simulink model "dfig"  (R2016a)
settings: Solver=VariableStepAuto  StartTime=0.0  StopTime=2  RelTol=1e-3
model workspace (MATLAB code in the model file):
  | Rs=1;
  | Vs=220;
  | fs=60;
  | p=2;
  | T=1e-4;
  | Ts=1e-5;
  | 
  | Ls=0.2010;
  | Rr=3.122;
  | Lr=0.2010;
  | Lm=0.1917;
  | 
  | Ps=3e3;
values from neighbouring files (symbols this model uses):
  dLm = delta(1)    [fitness.m]
  dRr = delta(2)    [fitness.m]
  Nu = 10    [fitness.m]
  Ny = 20    [fitness.m]
  StepFinal = [3,3]    [fitness.m]
  StepInit = [1,1]    [fitness.m]
  StepTime = [1,1.5]    [fitness.m]
  Variac = 120    [fitness.m]
  Wup = zeros(2*Nu,2*Nu)    [fitness.m]
  Wyp = zeros(2*Ny,2*Ny)    [fitness.m]
undefined symbols (not defined in the file or in its folder): DiscIntNeverNeededParam
libraries: powerlib x9, simulink x4, simulink_extras x3, dspfdesign x1
settings Model: Creator=Lucas  LastModifiedBy=lucas
settings SolverCC: ShapePreserveControl=EnableAll  ZeroCrossControl=DisableAll
settings DataIOCC: SignalLogging=off  DSMLogging=off

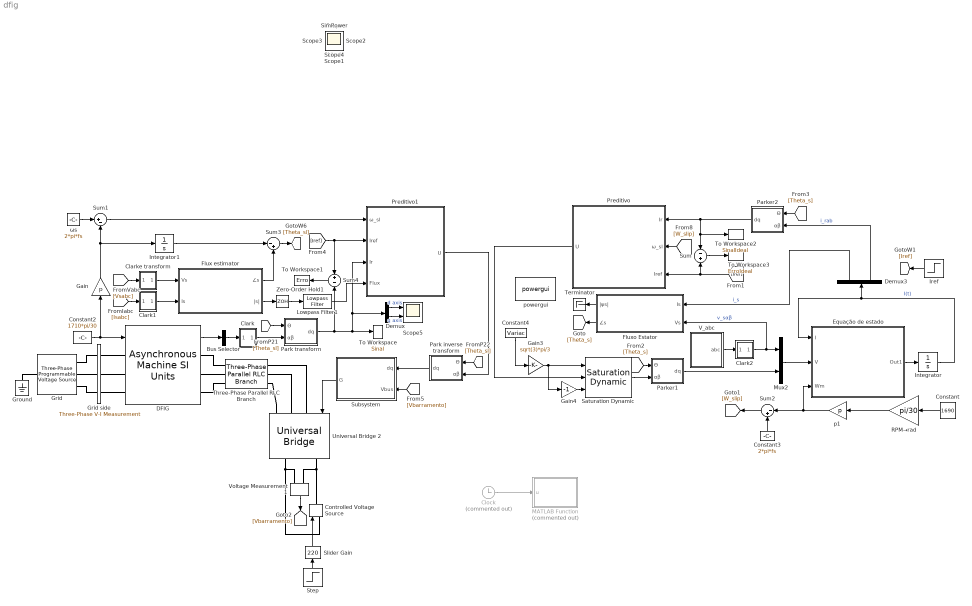
== system dfig ==
  Bus Selector : BusSelector  OutputSignals=Rotor measurements.Rotor current ir_a (A),Rotor measurements.Rotor current ir_b (A),Rotor measurements.Rotor current ir_c (A)  OutputAsBus=on
  Clark : Subsystem
      mask Display:
      | plot([0 1],[-1 0])
      | port_label('input',1,'3');
      | port_label('output', 1, '2', 'texmode', 'on')
  Clark1 : Subsystem
      mask Display:
      | plot([0 1],[-1 0])
      | port_label('input',1,'3');
      | port_label('output', 1, '2', 'texmode', 'on')
  Clark2 : Subsystem
      mask Display:
      | plot([0 1],[-1 0])
      | port_label('input',1,'3');
      | port_label('output', 1, '2', 'texmode', 'on')
  Clarke transform : Subsystem
      mask Display:
      | plot([0 1],[-1 0])
      | port_label('input',1,'3');
      | port_label('output', 1, '2', 'texmode', 'on')
  Clock : Clock  Commented=on
  Constant : Constant  Value=1690
  Constant2 : Constant  Value=1710*pi/30
      mask Display: disp('\fontsize{12}\omega_m','texmode','on')
  Constant3 : Constant  Value=2*pi*fs
      mask Display: disp('\omega_s','texmode','on')
  Constant4 : Constant  Value=Variac
  Controlled Voltage Source : powerlib/Electrical Sources/Controlled Voltage Source  Initialize=on  Source_Type=AC  Amplitude=0  Phase=0  Frequency=0  Measurements=None
  DFIG : powerlib/Machines/Asynchronous Machine SI Units  RotorType=Wound  PresetModel=No  MechanicalLoad=Speed w  ShowDetailedParameters=on  ReferenceFrame=Stationary  Units=SI  MeasurementBus=off  NominalParameters=[Ps Vs fs]  Stator=[Rs (Ls-Lm)]  Rotor=[Rr*(1+dRr/100) (Lr-Lm)]  Cage1=[0.4155 0.002066]  Cage2=[0.4168 0.0003495]  Lm=Lm*(1+dLm/100)  Mechanical=[0.05 0.005879 2]  PolePairs=p  InitialConditions=[0 0 0 0 0 0 0 0]  SimulateSaturation=off  Saturation=[14.03593122, 27.81365428, 53.79336849, 72.68890987, 97.98006896, 148.6815601, 215.7428561, 302.9841135, 428.7778367 ; 230, 322, 414, 460, 506, 552, 598, 644, 690]  LoadFlowParameters=1492000  TsPowergui=0  TsBlock=-1  IterativeModel=Trapezoidal non iterative  IterativeDiscreteModel=Trapezoidal non iterative  Pmec=0
  Demux : Demux  Outputs=2
  Demux3 : Demux  Outputs=2
  Equação de estado : Subsystem
      mask Display:
      | disp('\fontsize{16}A\cdotI(t)+B\cdotV(t)', 'texmode', 'on')
      | port_label('input', 1, 'I', 'texmode', 'on')
      | port_label('input', 2, 'V', 'texmode', 'on')
      | port_label('input', 3, '\omega_{m}', 'texmode', 'on')
      | port_label('output', 1, '\deltai(t)', 'texmode', 'on')
  Flux estimator : Subsystem
      mask Display:
      | disp('\fontsize{14}Flux Estimator', 'texmode', 'on')
      | port_label('output', 1, '\theta_s', 'texmode', 'on')
      | port_label('output', 2, '|\lambda_s|', 'texmode', 'on')
      | port_label('input', 1, 'v_s', 'texmode', 'on')
      | port_label('input', 2, 'i_s', 'texmode', 'on')
  Fluxo Estator : Subsystem
      mask Display:
      | disp('\fontsize{14}\lambda_s=\int(v_s-R_s\cdot i_s)dt', 'texmode', 'on')
      | port_label('output', 1, '|\lambda_s|', 'texmode', 'on')
      | port_label('output', 2, '\theta_s', 'texmode', 'on')
      | port_label('input', 2, 'v_s', 'texmode', 'on')
      | port_label('input', 1, 'i_s', 'texmode', 'on')
  Gain : Gain  Gain=p
  Gain3 : Gain  Gain=sqrt(3)*pi/3
  Gain4 : Gain  Gain=-1
  Grid : powerlib/Electrical Sources/Three-Phase Programmable Voltage Source  PositiveSequence="[220*sqrt(3)  0 60]"  VariationEntity=None  VariationType=Table of time-amplitude pairs  VariationTypeAlt=Step  VariationStep=0.5  VariationRate=[10]  VariationMagnitude=0.3  VariationFrequency=2  VariationTiming=[1 2]  VariationPhaseA=off  Amplitudes=[1 0.8 1.2 1.0]  TimeValues=[0 0.1 0.15 0.2]  HarmonicGeneration=off  HarmonicA=[3 0.2 -25 0]  HarmonicB=[2 0.15 35 2]  Timing="[0.05  3]"  BusType=swing  Pref=0  Qref=0  Qmin=-inf  Qmax=inf
  Grid side : powerlib/Measurements/Three-Phase V-I Measurement  VoltageMeasurement=phase-to-ground  SetLabelV=on  LabelV=Vsabc  Vpu=off  VpuLL=off  CurrentMeasurement=yes  SetLabelI=on  LabelI=Isabc  Ipu=off  Pbase=100e6  Vbase=500e3  OutputType=Complex  PhasorSimulation=off  PSBequivalent=0
  Ground : powerlib/Elements/Ground  LConnTagsString=a
  Integrator : Integrator  LimitOutput=on  UpperSaturationLimit=1e5  LowerSaturationLimit=-1e5
  Integrator1 : Integrator
  Iref : Step  Time=StepTime  Before=StepInit  After=StepFinal  SampleTime=0
  Lowpass Filter1 : dspfdesign/Lowpass Filter  FilterType=IIR  DesignForMinimumOrder=on  FilterOrder=50  PassbandFrequency=1e1  StopbandFrequency=1e2  PassbandRipple=0.1  StopbandAttenuation=80  InheritSampleRate=on  SampleRate=1e3  roundingMode=Floor  coeffsDataTypeStr=fixdt(1,16)  SimulateUsing=Interpreted execution
  MATLAB Function : MATLAB Function  Commented=on  TreatAsAtomicUnit=on
  Mux2 : Mux  Inputs=2
  Park inverse transform : Subsystem
      mask Display:
      | port_label('input', 2, 'x', 'texmode', 'on')
      | port_label('input', 1, '\theta', 'texmode', 'on')
      | port_label('output', 1, '\fontsize{14}xe^{ j\theta }', 'texmode', 'on')
  Park transform : Subsystem
      mask Display:
      | port_label('input', 2, 'x', 'texmode', 'on')
      | port_label('input', 1, '\theta', 'texmode', 'on')
      | port_label('output', 1, '\fontsize{14}xe^{ -j\theta} ', 'texmode', 'on')
  Parker1 : Subsystem
      mask Display:
      | port_label('input', 2, 'x', 'texmode', 'on')
      | port_label('input', 1, '\theta', 'texmode', 'on')
      | port_label('output', 1, '\fontsize{14}xe^{ j\theta }', 'texmode', 'on')
  Parker2 : Subsystem
      mask Display:
      | port_label('input', 2, 'x', 'texmode', 'on')
      | port_label('input', 1, '\theta', 'texmode', 'on')
      | port_label('output', 1, '\fontsize{14}xe^{ -j\theta }', 'texmode', 'on')
  Preditivo : Subsystem
      mask Display:
      | disp('\fontsize{14}Preditivo','texmode','on')
      | port_label('input', 1, 'i_{r dq} ', 'texmode', 'on')
      | port_label('input', 2, '\omega_{slip} ', 'texmode', 'on')
      | port_label('input', 3, 'i_{r ref}', 'texmode', 'on')
      | %port_label('input', 5, 'v_{r dq}', 'texmode', 'on')
      | port_label('output', 1, 'v_{r dq}', 'texmode', 'on')
  Preditivo1 : Subsystem
      mask Display:
      | disp('\fontsize{14}Predictive\newlineController','texmode','on')
      | port_label('input', 3, 'y(k)', 'texmode', 'on')
      | port_label('input', 4, '\lambda(k)', 'texmode', 'on')
      | port_label('input', 1, '\omega_{sl} ', 'texmode', 'on')
      | port_label('input', 2, 'y_{ref} (k)', 'texmode', 'on')
      | port_label('output', 1, 'u(k)', 'texmode', 'on')
  RPM→rad : Gain  Gain=pi/30
  Saturation Dynamic : simulink/Discontinuities/Saturation Dynamic  OutMin=[]  OutMax=[]  OutDataTypeStr=Inherit: Same as second input  OutDataType=fixdt(1, 16)  OutScaling=2^-10  DoSatur=off
  Scope5 : Scope  NumInputPorts=2
  Slider Gain : simulink/Math Operations/Slider Gain  low=1  gain=220  high=440
  Step : Step  Time=0  Before=1e-4  SampleTime=0
  Subsystem : Subsystem
      mask Display:
      | disp('\fontsize{14}SVPWM','texmode','on')
      | 
      | port_label('input', 1, 'dq', 'texmode', 'on')
      | port_label('input', 2, 'V_{bus}', 'texmode', 'on')
      | 
      | port_label('output', 1, 'G', 'texmode', 'on')
  Sum : Sum  Inputs=-|+
  Sum1 : Sum  Inputs=|+-
  Sum2 : Sum  Inputs=|-+
  Sum3 : Sum  Inputs=|-+
  Sum4 : Sum  Inputs=+|-
  Terminator : Terminator
  Three-Phase Parallel RLC Branch : powerlib/Elements/Three-Phase Parallel RLC Branch  LConnTagsString=A|B|C  RConnTagsString=A|B|C  BranchType=RL  Resistance=1  Inductance=1e-3  Capacitance=1e-6  Measurements=None
  To Workspace : ToWorkspace  VariableName=Sinal  SampleTime=-1
      mask Display: disp('\fontsize{12}i^{ s}_{r}','texmode','on')
  To Workspace1 : ToWorkspace  VariableName=Erro  SampleTime=-1
      mask Display: disp('Error')
  To Workspace2 : ToWorkspace  VariableName=SinalIdeal  SampleTime=-1
      mask Display: disp('Sinal')
  To Workspace3 : ToWorkspace  VariableName=ErroIdeal  SampleTime=-1
      mask Display: disp('Erro')
  Universal Bridge 2 : powerlib/Power Electronics/Universal Bridge  Arms=3  SnubberResistance=1e6  SnubberCapacitance=inf  Device=IGBT / Diodes  Ron=1e-4  Lon=0  ForwardVoltages="[  0  0  ]"  ForwardVoltage=0  GTOparameters=[ 10e-6 , 20e-6 ]  IGBTparameters=[ 1e-6 , 2e-6 ]*0  Measurements=None  Measurements_2=None  converterType=Rectifier
  V_abc : Subsystem  mask{A=Vs, f=fs}
      mask prompts: A "A - Amplitude (V)"; f "F - Frequência (Hz)"
      mask Display:
      | t = [0:pi/15:5*pi];
      | a = sin(t);
      | b = sin(t+2*pi/3);
      | c = sin(t-2*pi/3);
      | 
      | a(40:75)=NaN;
      | b(40:75)=NaN;
      | c(40:75)=NaN;
      | 
      | plot([0 0],[1.5 3.5]);
      | plot([0 2.8*pi],[2.5 2.5]);
      | plot(t,2.5+a);
      | 
      | port_label('output', 1, 'v_{abc} ', 'texmode', 'on')
      | 
      | plot([0 0],[-1 1]);
      | plot([0 2.8*pi],[0 0]);
      | plot(t,b);
      | 
      | plot([0 0],[-1.5 -3.5]);
      | plot([0 2.8*pi],[-2.5 -2.5]);
      | plot(t,-2.5+c);
  Voltage Measurement1 : powerlib/Measurements/Voltage Measurement  PhasorSimulation=off  OutputType=Complex  PSBequivalent=0
  Zero-Order Hold1 : ZeroOrderHold  SampleTime=T
  p1 : Gain  Gain=p
  powergui : powerlib/powergui  Priority=1  SimulationMode=Discrete  SolverType=Tustin/Backward Euler (TBE)  SampleTime=Ts  frequency=60  SPID=off  DisableSnubberDevices=off  DisableRonSwitches=off  DisableVfSwitches=off  SwTol=0  DisplayEquations=off  Interpol=off  ExternalGateDelay=off  methode=off  Ts=10  FunctionMessages=off  echomessages=off  HookPort=off  EnableUseOfTLC=off  x0status=blocks  frequencyindice=0  Pbase=100e6  ErrMax=1e-4  Iterations=50  UnitsV=kV  UnitsW=MW  buscounter=0  RestoreLinks=warning  ResistiveCurrentMeasurement=off  Frange=[0:2:500]  Ylog=off  Xlog=on  ShowGrid=off  save=off  variable=ZData  structure=0  ZoomFFT=off  StartTime=0.0  cycles=1  DisplayStyle=1  fundamental=60  FreqAxis=off  MaxFrequency=1000  frequencyindicesteady=1  RmsSteady=1  display=off
  ωs : Constant  Value=2*pi*fs
      mask Display: disp('\fontsize{12}\omega_s','texmode','on')
  Ideal : Scope
  Scope{,1..4} (5 alike) : Scope
  SimPower : Scope
  wires:
  Constant2/1 -> DFIG/1, Gain/1
  Clark/1(αβ) -> Park transform/2(αβ)
  [Theta_sl] -> Park transform/1(Θ)
  Clarke transform/1(αβ) -> Flux estimator/1(Vs)
  Clark1/1(αβ) -> Flux estimator/2(Is)
  [Vsabc] -> Clarke transform/1(abc)
  [Isabc] -> Clark1/1(abc)
  Gain/1 -> Sum1/2, Integrator1/1
  Integrator1/1 -> Sum3/1
  Flux estimator/1(∠s) -> Sum3/2
  Sum3/1 -> [Theta_sl]
  ωs/1 -> Sum1/1
  Sum1/1 -> Preditivo1/1(" ω_sl")
  [Theta_sl] -> Park inverse transform/1(Θ)
  Preditivo1/1(U) -> Park inverse transform/2(αβ)
  Sum4/1 -> To Workspace1/1
  Integrator/1 -> Equação de estado/1(I), Demux3/1  "I(t)"
  V_abc/1(abc) -> Clark2/1(abc)
  Equação de estado/1(Out1) -> Integrator/1
  Clark2/1(αβ) -> Fluxo Estator/2(Vs), Mux2/1  "v_sαβ"
  Mux2/1 -> Equação de estado/2(V)
  Constant/1 -> RPM→rad/1
  Demux3/1 -> Fluxo Estator/1(Is)  "i_s"
  Demux3/2 -> Parker2/2(αβ)  "i_rab"
  Constant3/1 -> Sum2/2
  Sum2/1 -> [W_slip]
  [Iref] -> Preditivo/3(Iref), Sum/2
  [W_slip] -> Preditivo/2(" ω_sl")
  p1/1 -> Sum2/1, Equação de estado/3(Wm)
  [Theta_s] -> Parker2/1(Θ)
  Fluxo Estator/1(|ψs|) -> Terminator/1
  Sum/1 -> To Workspace3/1
  Parker2/1(dq) -> To Workspace2/1, Sum/1, Preditivo/1(Ir)
  [Theta_s] -> Parker1/1(Θ)
  Parker1/1(dq) -> Mux2/2
  Preditivo/1(U) -> Saturation Dynamic/2
  Gain3/1 -> Gain4/1, Saturation Dynamic/1
  Gain4/1 -> Saturation Dynamic/3
  Constant4/1 -> Gain3/1
  Saturation Dynamic/1 -> Parker1/2(αβ)
  Fluxo Estator/2(∠s) -> [Theta_s]
  RPM→rad/1 -> p1/1
  Iref/1 -> [Iref]
  [Iref] -> Sum4/1, Preditivo1/2(Iref)
  Park inverse transform/1(dq) -> Subsystem/1(dq)
  Subsystem/1(G) -> Universal Bridge 2/1
  DFIG/1 -> Bus Selector/1
  Bus Selector/1 -> Clark/1(abc)
  Flux estimator/2(|s|) -> Zero-Order Hold1/1
  Voltage Measurement1/1 -> [Vbarramento]
  Slider Gain/1 -> Controlled Voltage Source/1
  [Vbarramento] -> Subsystem/2(Vbus)
  Zero-Order Hold1/1 -> Lowpass Filter1/1
  Lowpass Filter1/1 -> Preditivo1/4(Flux)
  Demux/1 -> Scope5/1  "d axis"
  Demux/2 -> Scope5/2  "q axis"
  Clock/1 -> MATLAB Function/1(u)
  Step/1 -> Slider Gain/1
  Park transform/1(dq) -> To Workspace/1, Preditivo1/3(Ir), Demux/1, Sum4/2
  connections:
  Grid/LConn1 -- Ground/LConn1
  Grid/RConn3 -- Grid side/LConn3
  Grid side/RConn3 -- DFIG/LConn3
  Grid side/RConn1 -- DFIG/LConn1
  Grid side/RConn2 -- DFIG/LConn2
  Grid side/LConn1 -- Grid/RConn1
  Grid side/LConn2 -- Grid/RConn2
  Controlled Voltage Source/LConn1 -- Voltage Measurement1/LConn2 -- Universal Bridge 2/RConn2
  Controlled Voltage Source/RConn1 -- Voltage Measurement1/LConn1 -- Universal Bridge 2/RConn1
  Three-Phase Parallel RLC Branch/RConn1 -- Universal Bridge 2/LConn1
  Universal Bridge 2/LConn2 -- Three-Phase Parallel RLC Branch/RConn2
  Universal Bridge 2/LConn3 -- Three-Phase Parallel RLC Branch/RConn3
  Three-Phase Parallel RLC Branch/LConn1 -- DFIG/RConn1
  Three-Phase Parallel RLC Branch/LConn2 -- DFIG/RConn2
  Three-Phase Parallel RLC Branch/LConn3 -- DFIG/RConn3

== system dfig/Clark ==
  abc : Inport
  Mux : Mux  Inputs=2
  xα : Fcn  Expr=2/3*(u(1)-u(2)/2-u(3)/2)
  xβ : Fcn  Expr=(u(2) - u(3))/sqrt(3)
  αβ : Outport
  wires:
  abc/1 -> xα/1, xβ/1
  Mux/1 -> αβ/1
  xα/1 -> Mux/1
  xβ/1 -> Mux/2

== system dfig/Clark1 ==
  abc : Inport
  Mux : Mux  Inputs=2
  xα : Fcn  Expr=2/3*(u(1)-u(2)/2-u(3)/2)
  xβ : Fcn  Expr=(u(2) - u(3))/sqrt(3)
  αβ : Outport
  wires:
  abc/1 -> xα/1, xβ/1
  Mux/1 -> αβ/1
  xα/1 -> Mux/1
  xβ/1 -> Mux/2

== system dfig/Clark2 ==
  abc : Inport
  Mux : Mux  Inputs=2
  xα : Fcn  Expr=2/3*(u(1)-u(2)/2-u(3)/2)
  xβ : Fcn  Expr=(u(2) - u(3))/sqrt(3)
  αβ : Outport
  wires:
  abc/1 -> xα/1, xβ/1
  Mux/1 -> αβ/1
  xα/1 -> Mux/1
  xβ/1 -> Mux/2

== system dfig/Clarke transform ==
  abc : Inport
  Mux : Mux  Inputs=2
  xα : Fcn  Expr=2/3*(u(1)-u(2)/2-u(3)/2)
  xβ : Fcn  Expr=(u(2) - u(3))/sqrt(3)
  αβ : Outport
  wires:
  abc/1 -> xα/1, xβ/1
  Mux/1 -> αβ/1
  xα/1 -> Mux/1
  xβ/1 -> Mux/2

== system dfig/Equação de estado ==
  I : Inport
  V : Inport  Port=2
  Wm : Inport  Port=3
  Demux : Demux
  Demux1 : Demux
  Espaço de estado : MATLAB Function  TreatAsAtomicUnit=on
  Out1 : Outport
  wires:
  Espaço de estado/1(dI) -> Out1/1
  Demux/1 -> Espaço de estado/1(I_as)
  Demux/2 -> Espaço de estado/2(I_bs)
  Demux/3 -> Espaço de estado/3(I_ar)
  Demux/4 -> Espaço de estado/4(I_br)
  I/1 -> Demux/1
  Demux1/1 -> Espaço de estado/5(V_as)
  Demux1/2 -> Espaço de estado/6(V_bs)
  Demux1/3 -> Espaço de estado/7(V_ar)
  Demux1/4 -> Espaço de estado/8(V_br)
  V/1 -> Demux1/1
  Wm/1 -> Espaço de estado/9(Wm)

== system dfig/Flux estimator ==
  Vs : Inport
  Is : Inport  Port=2
  Cartesian to Polar : simulink_extras/Transformations/Cartesian to Polar
  Demux : Demux  Outputs=2
  Gain : Gain  Gain=Rs
  Integrator : Integrator
  Sum : Sum  Inputs=|+-
  ∠s : Outport
  |s| : Outport  Port=2
  wires:
  Integrator/1 -> Demux/1
  Demux/1 -> Cartesian to Polar/1
  Demux/2 -> Cartesian to Polar/2
  Cartesian to Polar/1 -> |s|/1
  Gain/1 -> Sum/2
  Is/1 -> Gain/1
  Vs/1 -> Sum/1
  Sum/1 -> Integrator/1
  Cartesian to Polar/2 -> ∠s/1

== system dfig/Fluxo Estator ==
  Is : Inport
  Vs : Inport  Port=2
  Cartesian to Polar : simulink_extras/Transformations/Cartesian to Polar
  Demux : Demux  Outputs=2
  Gain : Gain  Gain=Rs
  Integrator : Integrator
  Sum : Sum  Inputs=|+-
  |ψs| : Outport
  ∠s : Outport  Port=2
  wires:
  Integrator/1 -> Demux/1
  Demux/1 -> Cartesian to Polar/1
  Demux/2 -> Cartesian to Polar/2
  Cartesian to Polar/1 -> |ψs|/1
  Gain/1 -> Sum/2
  Is/1 -> Gain/1
  Vs/1 -> Sum/1
  Sum/1 -> Integrator/1
  Cartesian to Polar/2 -> ∠s/1

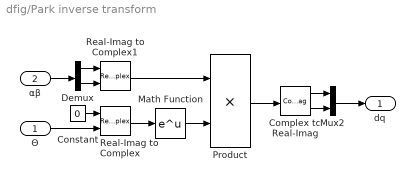
== system dfig/Park inverse transform ==
  Θ : Inport
  αβ : Inport  Port=2
  Complex to Real-Imag : ComplexToRealImag
  Constant : Constant  Value=0
  Demux : Demux  Outputs=2
  Math Function : Math  SaturateOnIntegerOverflow=on
  Mux2 : Mux  Inputs=2
  Product : Product
  Real-Imag to Complex : RealImagToComplex
  Real-Imag to Complex1 : RealImagToComplex
  dq : Outport
  wires:
  Real-Imag to Complex/1 -> Math Function/1
  Θ/1 -> Real-Imag to Complex/2
  Constant/1 -> Real-Imag to Complex/1
  Demux/2 -> Real-Imag to Complex1/2
  Demux/1 -> Real-Imag to Complex1/1
  αβ/1 -> Demux/1
  Math Function/1 -> Product/2
  Real-Imag to Complex1/1 -> Product/1
  Product/1 -> Complex to Real-Imag/1
  Complex to Real-Imag/1 -> Mux2/1
  Complex to Real-Imag/2 -> Mux2/2
  Mux2/1 -> dq/1

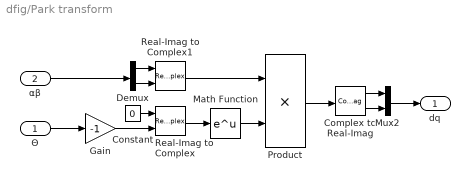
== system dfig/Park transform ==
  Θ : Inport
  αβ : Inport  Port=2
  Complex to Real-Imag : ComplexToRealImag
  Constant : Constant  Value=0
  Demux : Demux  Outputs=2
  Gain : Gain  Gain=-1
  Math Function : Math  SaturateOnIntegerOverflow=on
  Mux2 : Mux  Inputs=2
  Product : Product
  Real-Imag to Complex : RealImagToComplex
  Real-Imag to Complex1 : RealImagToComplex
  dq : Outport
  wires:
  Real-Imag to Complex/1 -> Math Function/1
  Θ/1 -> Gain/1
  Constant/1 -> Real-Imag to Complex/1
  Demux/2 -> Real-Imag to Complex1/2
  Demux/1 -> Real-Imag to Complex1/1
  αβ/1 -> Demux/1
  Math Function/1 -> Product/2
  Real-Imag to Complex1/1 -> Product/1
  Product/1 -> Complex to Real-Imag/1
  Complex to Real-Imag/1 -> Mux2/1
  Complex to Real-Imag/2 -> Mux2/2
  Mux2/1 -> dq/1
  Gain/1 -> Real-Imag to Complex/2

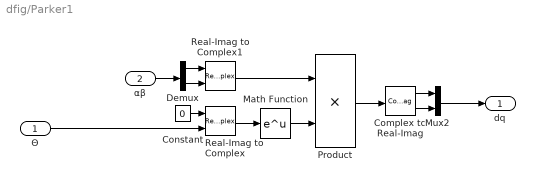
== system dfig/Parker1 ==
  Θ : Inport
  αβ : Inport  Port=2
  Complex to Real-Imag : ComplexToRealImag
  Constant : Constant  Value=0
  Demux : Demux  Outputs=2
  Math Function : Math  SaturateOnIntegerOverflow=on
  Mux2 : Mux  Inputs=2
  Product : Product
  Real-Imag to Complex : RealImagToComplex
  Real-Imag to Complex1 : RealImagToComplex
  dq : Outport
  wires:
  Real-Imag to Complex/1 -> Math Function/1
  Constant/1 -> Real-Imag to Complex/1
  Demux/2 -> Real-Imag to Complex1/2
  Demux/1 -> Real-Imag to Complex1/1
  αβ/1 -> Demux/1
  Math Function/1 -> Product/2
  Real-Imag to Complex1/1 -> Product/1
  Product/1 -> Complex to Real-Imag/1
  Complex to Real-Imag/1 -> Mux2/1
  Complex to Real-Imag/2 -> Mux2/2
  Mux2/1 -> dq/1
  Θ/1 -> Real-Imag to Complex/2

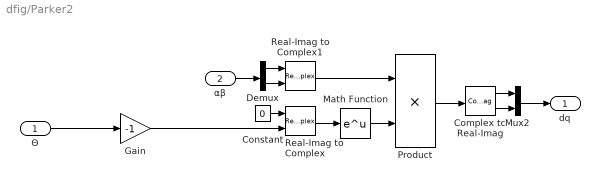
== system dfig/Parker2 ==
  Θ : Inport
  αβ : Inport  Port=2
  Complex to Real-Imag : ComplexToRealImag
  Constant : Constant  Value=0
  Demux : Demux  Outputs=2
  Gain : Gain  Gain=-1
  Math Function : Math  SaturateOnIntegerOverflow=on
  Mux2 : Mux  Inputs=2
  Product : Product
  Real-Imag to Complex : RealImagToComplex
  Real-Imag to Complex1 : RealImagToComplex
  dq : Outport
  wires:
  Real-Imag to Complex/1 -> Math Function/1
  Θ/1 -> Gain/1
  Constant/1 -> Real-Imag to Complex/1
  Demux/2 -> Real-Imag to Complex1/2
  Demux/1 -> Real-Imag to Complex1/1
  αβ/1 -> Demux/1
  Math Function/1 -> Product/2
  Real-Imag to Complex1/1 -> Product/1
  Product/1 -> Complex to Real-Imag/1
  Complex to Real-Imag/1 -> Mux2/1
  Complex to Real-Imag/2 -> Mux2/2
  Mux2/1 -> dq/1
  Gain/1 -> Real-Imag to Complex/2

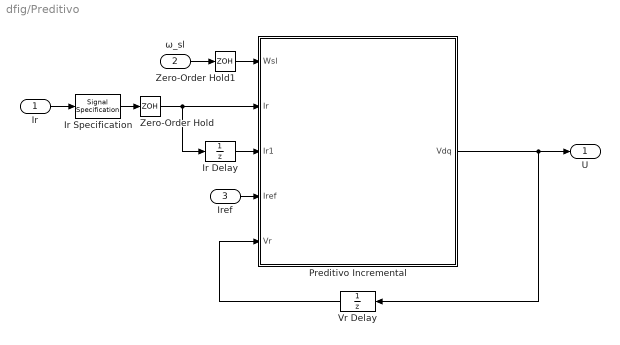
== system dfig/Preditivo ==
  Ir : Inport
  " ω_sl" : Inport  Port=2
  Iref : Inport  Port=3
  Ir Delay : UnitDelay  SampleTime=-1
  Ir Specification : SignalSpecification  Dimensions=2
  Preditivo Incremental : MATLAB Function  TreatAsAtomicUnit=on  SystemSampleTime=T
  Vr Delay : UnitDelay  SampleTime=-1
  Zero-Order Hold : ZeroOrderHold  SampleTime=T
  Zero-Order Hold1 : ZeroOrderHold  SampleTime=T
  U : Outport
  wires:
  Ir/1 -> Ir Specification/1
  " ω_sl"/1 -> Zero-Order Hold1/1
  Iref/1 -> Preditivo Incremental/4(Iref)
  Zero-Order Hold1/1 -> Preditivo Incremental/1(Wsl)
  Vr Delay/1 -> Preditivo Incremental/5(Vr)
  Zero-Order Hold/1 -> Ir Delay/1, Preditivo Incremental/2(Ir)
  Ir Delay/1 -> Preditivo Incremental/3(Ir1)
  Ir Specification/1 -> Zero-Order Hold/1
  Preditivo Incremental/1(Vdq) -> U/1, Vr Delay/1

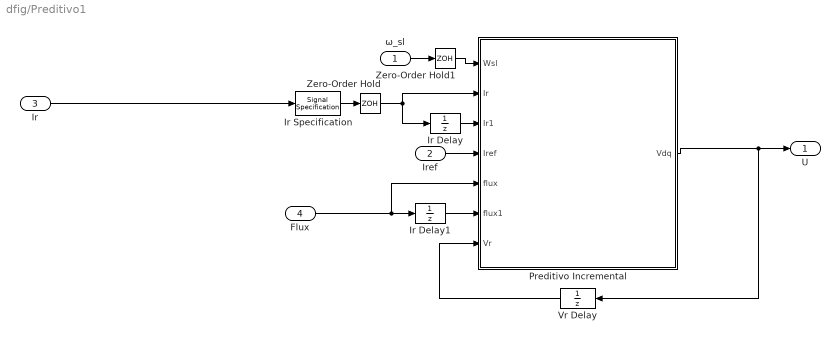
== system dfig/Preditivo1 ==
  " ω_sl" : Inport
  Iref : Inport  Port=2
  Ir : Inport  Port=3
  Flux : Inport  Port=4
  Ir Delay : UnitDelay  SampleTime=-1
  Ir Delay1 : UnitDelay  SampleTime=-1
  Ir Specification : SignalSpecification  Dimensions=2
  Preditivo Incremental : MATLAB Function  TreatAsAtomicUnit=on  SystemSampleTime=T
  Vr Delay : UnitDelay  SampleTime=-1
  Zero-Order Hold : ZeroOrderHold  SampleTime=T
  Zero-Order Hold1 : ZeroOrderHold  SampleTime=T
  U : Outport
  wires:
  Ir/1 -> Ir Specification/1
  " ω_sl"/1 -> Zero-Order Hold1/1
  Iref/1 -> Preditivo Incremental/4(Iref)
  Zero-Order Hold1/1 -> Preditivo Incremental/1(Wsl)
  Vr Delay/1 -> Preditivo Incremental/7(Vr)
  Zero-Order Hold/1 -> Ir Delay/1, Preditivo Incremental/2(Ir)
  Ir Delay/1 -> Preditivo Incremental/3(Ir1)
  Ir Specification/1 -> Zero-Order Hold/1
  Preditivo Incremental/1(Vdq) -> U/1, Vr Delay/1
  Ir Delay1/1 -> Preditivo Incremental/6(flux1)
  Flux/1 -> Preditivo Incremental/5(flux), Ir Delay1/1

== system dfig/Subsystem ==
  dq : Inport
  Vbus : Inport  Port=2
  Rampa : Subsystem  mask{Ftri_=1/T, Ts=Ts}
      mask prompts: Ftri_ "Ftri - Frequência da portadora"; Ts "Ts - Periodo de amostragem"
      mask Display:
      | t = [0,0.25,0.25,0.5,0.5];
      | a = [0,0.75,0,0.75,0];
      | plot(0.3+t,a+0.125);
      | 
      | port_label('output',1,'v_{trig} ','texmode','on')
      | port_label('output',2,'v_{tri} ','texmode','on')
  SVPWM : Subsystem
      mask Display:
      | disp('\fontsize{14}SVPWM','texmode','on')
      | port_label('input',1,'dq','texmode','on')
      | port_label('input',2,'v_{trig}','texmode','on')
      | port_label('input',3,'v_{tri}','texmode','on')
      | port_label('input',4,'v_{bus}','texmode','on')
      | port_label('output',1,'G','texmode','on')
  G : Outport
  wires:
  Vbus/1 -> SVPWM/4(Vdc)
  Rampa/1(Trigger) -> SVPWM/2(Trigger)
  Rampa/2(Vtri) -> SVPWM/3(Vtri)
  dq/1 -> SVPWM/1(dq)
  SVPWM/1(G) -> G/1

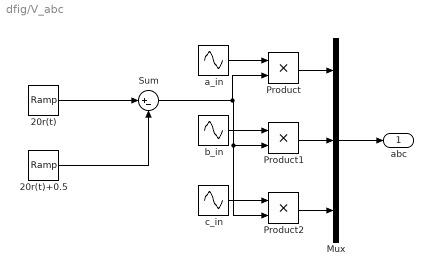
== system dfig/V_abc ==
  20r(t) : simulink/Sources/Ramp  slope=20  start=0  X0=0
  20r(t)+0.5 : simulink/Sources/Ramp  slope=20  start=0.05  X0=0
  Mux : Mux  Inputs=3
  Product : Product
  Product1 : Product
  Product2 : Product
  Sum : Sum  Inputs=|+-
  a_in : Sin  Amplitude=A*2^0.5  Frequency=2*pi*f  SampleTime=0
  b_in : Sin  Amplitude=A*2^0.5  Frequency=2*pi*f  Phase=-2*pi/3  SampleTime=0
  c_in : Sin  Amplitude=A*2^0.5  Frequency=2*pi*f  Phase=2*pi/3  SampleTime=0
  abc : Outport
  wires:
  c_in/1 -> Product2/1
  Sum/1 -> Product2/2, Product1/2, Product/2
  b_in/1 -> Product1/1
  a_in/1 -> Product/1
  Mux/1 -> abc/1
  Product1/1 -> Mux/2
  Product/1 -> Mux/1
  Product2/1 -> Mux/3
  20r(t)/1 -> Sum/1
  20r(t)+0.5/1 -> Sum/2

== system dfig/Subsystem/Rampa ==
  Constant : Constant  Value=Ftri_
  Constant3 : Constant
  Discrete-Time Integrator : DiscreteIntegrator  ExternalReset=rising  InitialConditionSetting=State (most efficient)  SampleTime=Ts  ICPrevOutput=DiscIntNeverNeededParam  ICPrevScaledInput=DiscIntNeverNeededParam
  Relational Operator1 : RelationalOperator  InputSameDT=on
  Unit Delay1 : UnitDelay  SampleTime=Ts
  Trigger : Outport
  Vtri : Outport  Port=2
  wires:
  Discrete-Time Integrator/1 -> Vtri/1, Relational Operator1/1
  Constant/1 -> Discrete-Time Integrator/1
  Constant3/1 -> Relational Operator1/2
  Unit Delay1/1 -> Trigger/1, Discrete-Time Integrator/2
  Relational Operator1/1 -> Unit Delay1/1

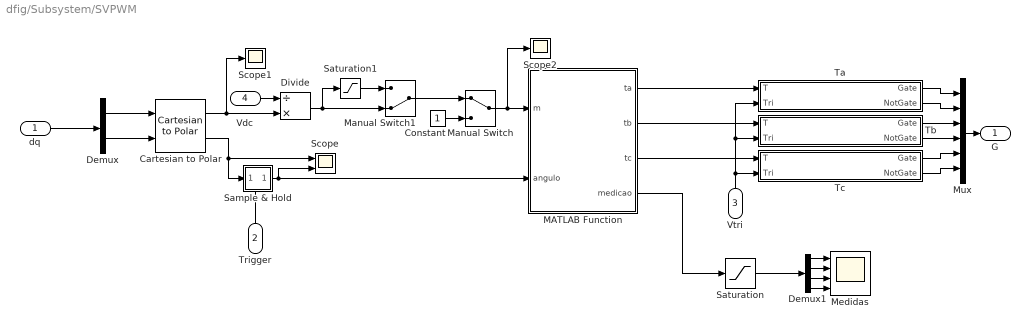
== system dfig/Subsystem/SVPWM ==
  dq : Inport
  Trigger : Inport  Port=2
  Vtri : Inport  Port=3
  Vdc : Inport  Port=4
  Cartesian to Polar : simulink_extras/Transformations/Cartesian to Polar
  Constant : Constant
  Demux : Demux  Outputs=2
  Demux1 : Demux
  Divide : Product  Inputs=/*
  MATLAB Function : MATLAB Function  TreatAsAtomicUnit=on
  Manual Switch : ManualSwitch
  Manual Switch1 : ManualSwitch  CurrentSetting=0
  Medidas : Scope  NumInputPorts=4
  Mux : Mux  Inputs=6
  Sample & Hold : Subsystem
      mask Display: disp('S/H');
  Saturation : Saturate  UpperLimit=2
  Saturation1 : Saturate  UpperLimit=1  LowerLimit=0
  Scope : Scope  NumInputPorts=2
  Scope1 : Scope
  Scope2 : Scope
  Ta : Subsystem
      mask Display:
      | disp('Selecionador\ndo Gate');
      | port_label('input',1,'t','texmode','on')
      | port_label('input',2,'V_{tri}','texmode','on')
      | port_label('output',1,'G','texmode','on')
      | port_label('output',2,'G_{NOT}','texmode','on')
  Tb : Subsystem
      mask Display:
      | disp('Selecionador\ndo Gate');
      | port_label('input',1,'t','texmode','on')
      | port_label('input',2,'V_{tri}','texmode','on')
      | port_label('output',1,'G','texmode','on')
      | port_label('output',2,'G_{NOT}','texmode','on')
  Tc : Subsystem
      mask Display:
      | disp('Selecionador\ndo Gate');
      | port_label('input',1,'t','texmode','on')
      | port_label('input',2,'V_{tri}','texmode','on')
      | port_label('output',1,'G','texmode','on')
      | port_label('output',2,'G_{NOT}','texmode','on')
  G : Outport
  wires:
  Sample & Hold/1(Out) -> MATLAB Function/2(angulo), Scope/2
  dq/1 -> Demux/1
  MATLAB Function/4(medicao) -> Saturation/1
  Demux/2 -> Cartesian to Polar/2
  Demux/1 -> Cartesian to Polar/1
  MATLAB Function/3(tc) -> Tc/1(T)
  MATLAB Function/2(tb) -> Tb/1(T)
  MATLAB Function/1(ta) -> Ta/1(T)
  Demux1/2 -> Medidas/2
  Demux1/4 -> Medidas/4
  Demux1/3 -> Medidas/3
  Demux1/1 -> Medidas/1
  Trigger/1 -> Sample & Hold/Trigger
  Vtri/1 -> Ta/2(Tri), Tb/2(Tri), Tc/2(Tri)
  Ta/1(Gate) -> Mux/1
  Ta/2(NotGate) -> Mux/2
  Tb/1(Gate) -> Mux/3
  Tb/2(NotGate) -> Mux/4
  Tc/1(Gate) -> Mux/5
  Tc/2(NotGate) -> Mux/6
  Mux/1 -> G/1
  Saturation/1 -> Demux1/1
  Cartesian to Polar/2 -> Sample & Hold/1(In), Scope/1
  Manual Switch/1 -> Scope2/1, MATLAB Function/1(m)
  Cartesian to Polar/1 -> Scope1/1, Divide/2
  Vdc/1 -> Divide/1
  Constant/1 -> Manual Switch/2
  Divide/1 -> Saturation1/1, Manual Switch1/2
  Saturation1/1 -> Manual Switch1/1
  Manual Switch1/1 -> Manual Switch/1

== system dfig/Subsystem/SVPWM/Sample & Hold ==
  In : Inport
  Trigger : TriggerPort  VariantControl=Variant  PortDimensions=1
  Out : Outport
  wires:
  In/1 -> Out/1

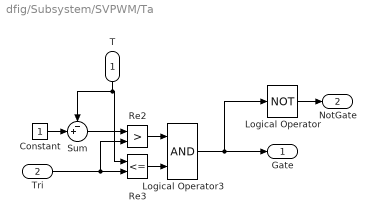
== system dfig/Subsystem/SVPWM/Ta ==
  T : Inport
  Tri : Inport  Port=2
  Constant : Constant
  Logical Operator : Logic  Operator=NOT  AllPortsSameDT=off  OutDataTypeStr=boolean
  Logical Operator3 : Logic  AllPortsSameDT=off  OutDataTypeStr=boolean
  Re2 : RelationalOperator  Operator=>  OutDataTypeStr=boolean
  Re3 : RelationalOperator  Operator=<=  OutDataTypeStr=boolean
  Sum : Sum  Inputs=-+|
  Gate : Outport
  NotGate : Outport  Port=2
  wires:
  T/1 -> Sum/1, Re3/1
  Constant/1 -> Sum/2
  Tri/1 -> Re2/2, Re3/2
  Re2/1 -> Logical Operator3/1
  Re3/1 -> Logical Operator3/2
  Sum/1 -> Re2/1
  Logical Operator3/1 -> Logical Operator/1, Gate/1
  Logical Operator/1 -> NotGate/1

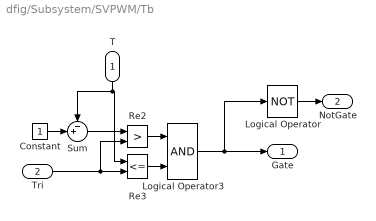
== system dfig/Subsystem/SVPWM/Tb ==
  T : Inport
  Tri : Inport  Port=2
  Constant : Constant
  Logical Operator : Logic  Operator=NOT  AllPortsSameDT=off  OutDataTypeStr=boolean
  Logical Operator3 : Logic  AllPortsSameDT=off  OutDataTypeStr=boolean
  Re2 : RelationalOperator  Operator=>  OutDataTypeStr=boolean
  Re3 : RelationalOperator  Operator=<=  OutDataTypeStr=boolean
  Sum : Sum  Inputs=-+|
  Gate : Outport
  NotGate : Outport  Port=2
  wires:
  T/1 -> Sum/1, Re3/1
  Constant/1 -> Sum/2
  Tri/1 -> Re2/2, Re3/2
  Re2/1 -> Logical Operator3/1
  Re3/1 -> Logical Operator3/2
  Sum/1 -> Re2/1
  Logical Operator3/1 -> Logical Operator/1, Gate/1
  Logical Operator/1 -> NotGate/1

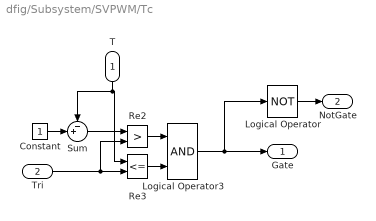
== system dfig/Subsystem/SVPWM/Tc ==
  T : Inport
  Tri : Inport  Port=2
  Constant : Constant
  Logical Operator : Logic  Operator=NOT  AllPortsSameDT=off  OutDataTypeStr=boolean
  Logical Operator3 : Logic  AllPortsSameDT=off  OutDataTypeStr=boolean
  Re2 : RelationalOperator  Operator=>  OutDataTypeStr=boolean
  Re3 : RelationalOperator  Operator=<=  OutDataTypeStr=boolean
  Sum : Sum  Inputs=-+|
  Gate : Outport
  NotGate : Outport  Port=2
  wires:
  T/1 -> Sum/1, Re3/1
  Constant/1 -> Sum/2
  Tri/1 -> Re2/2, Re3/2
  Re2/1 -> Logical Operator3/1
  Re3/1 -> Logical Operator3/2
  Sum/1 -> Re2/1
  Logical Operator3/1 -> Logical Operator/1, Gate/1
  Logical Operator/1 -> NotGate/1

== matlab function dfig/Equação de estado/Espaço de estado ==
  data: I_as input; dI output; I_bs input; I_ar input; I_br input; V_as input; V_bs input; V_ar input; V_br input; Wm input; Rs parameter; Ls parameter; Rr parameter; Lr parameter; Lm parameter; dLm parameter; dRr parameter
function dI = espaco_estado(I_as,I_bs,I_ar,I_br,V_as,V_bs,V_ar,V_br,Wm,Rs, Ls, Rr, Lr, Lm,dLm, dRr)
Rr=Rr*(1+dRr/100);
Lm=Lm*(1+dLm/100);
Ls=Ls+Lm*dLm/100;
Lr=Lr+Lm*dLm/100;
% I = [I_αs,I_βs, I_αr, I_βr]
I = [I_as;I_bs;I_ar;I_br];
% V = [V_αs,V_βs, V_αr, V_βr] [Rs Ls Rr Lr Lm]
V = [V_as;V_bs;V_ar;V_br];
A = [-Rs*Lr,   Wm*Lm^2,   Rr*Lm,     Wm*Lm*Lr;
     -Wm*Lm^2, -Rs*Lr,    -Wm*Lm*Lr, Rr*Lm;
     Rs*Lm,    -Wm*Ls*Lm, -Rr*Ls,    -Wm*Lr*Ls;
     Wm*Ls*Lm, Rs*Lm,     Wm*Lr*Ls,  -Rr*Ls];
 
B = [Lr,  0,  -Lm, 0;
     0,   Lr,  0,   -Lm;
     -Lm, 0,   Ls, 0;
     0,   -Lm, 0,  Ls];
S = 1-Lm^2/(Ls*Lr);
K = 1/(S*Ls*Lr);



A = K*A;
B = K*B;

dI = A*I+B*V;

== matlab function dfig/Subsystem/SVPWM/MATLAB Function ==
  data: m input; angulo input; ta output; tb output; tc output; medicao output size=[1 4]
function [ta,tb,tc,medicao] = fcn(m,angulo)
%Procurar setor
if (angulo >=0) && (angulo < pi/3)
    setor = 1;
elseif (angulo >=pi/3) && (angulo < 2*pi/3)
    setor = 2;
elseif (angulo >=2*pi/3) && (angulo < pi)
    setor = 3;
elseif (angulo >=-pi) && (angulo < -2*pi/3)
    setor = 4;
elseif (angulo >=-2*pi/3) && (angulo < -pi/3)
    setor = 5;
else
    setor = 6;
end
theta_l=pi/3*setor-angulo;
t1=m*sin(theta_l)/sqrt(3);
t2=m*sin(pi/3-theta_l)/sqrt(3);
t0=0.5-t1-t2;
if t0<0
   t1=t1/(t1+t2);
   t2=t2/(t1+t2);
   t0=0;
end
t0=t0/2;
switch setor
    case 1
        ta=t0;
        tb=t0+t1;
        tc=t0+t1+t2;
    case 2
        ta=t0+t2;
        tb=t0;
        tc=t0+t1+t2;
    case 3
        ta=t0+t1+t2;
        tb=t0;
        tc=t0+t1;
    case 4
        ta=t0+t1+t2;
        tb=t0+t2;
        tc=t0;
    case 5
        ta=t0+t1;
        tb=t0+t1+t2;
        tc=t0;
    otherwise
        ta=t0;
        tb=t0+t1+t2;
        tc=t0+t2;
end
medicao=[t0,t1,t2,m];

== matlab function dfig/Preditivo/Preditivo Incremental ==
  data: Wsl input; Ir input; Ir1 input; Iref input; Ls parameter; Lr parameter; Rr parameter; Lm parameter; T parameter; Nu parameter; Ny parameter; Vdq output; Wyp parameter; Wup parameter; Vr input
function Vdq  = fcn(Wsl,Ir, Ir1,Iref,Ls, Lr, Rr, Lm, T, Nu, Ny, Wyp, Wup, Vr)
assert (Ny <= 100);
assert (Nu <= 100);

%Variáveis auxiliares

Sigma = 1-Lm^2/(Ls*Lr);

%Entradas
eps = [Ir(1)-Ir1(1);Ir(2)-Ir1(2);Ir(1);Ir(2)];


%Matrizes de estado discretizadas
A = [1-Rr*T/(Sigma*Lr),       Wsl*T;
          -Wsl*T,        1-Rr*T/(Sigma*Lr)];

B = [T/(Sigma*Lr),      0;
          0,        T/(Sigma*Lr)];
      
C = eye(2);


Aa=[A,zeros(2); C*A,eye(2)];

Ba = [B;C*B];

Ca = [zeros(2), eye(2)];
 
%Inicialização de matrizes
Ap = zeros(2*Ny,4);
Bp = zeros(2*Ny,2*Nu);

Refp = zeros(2*Ny,1);


%Cálculo das matrizes
for i=1:Ny
    Ap((i-1)*2+1:i*2,1:4)= Ca*Aa^i;
    Refp((i-1)*2+1:i*2,1)=Iref;
    for j=1:i
        if j<=Nu
            Bp((i-1)*2+1:i*2,(j-1)*2+1:j*2)=Ca*Aa^(i-j)*Ba;
        end
    end
end
%Minimização

dU = (Bp.'*Wyp*Bp+Wup)\(Bp.'*Wyp*(Refp-Ap*eps));
% 164.3*Ird1 - 306.4*Ird + 142.1*Irefd - 0.0304*Irefq - 0.3686*Irq + 0.399*Irq1
%   36.95*Ird + 14.14*Ird1 - 51.09*Irefd + 93.76*Irefq - 229.9*Irq + 136.1*Irq1
Vdq = Vr + dU(1:2,1);

== matlab function dfig/Preditivo1/Preditivo Incremental ==
  data: Wsl input; Ir input; Ir1 input; Iref input; Ls parameter; Lr parameter; Rr parameter; Lm parameter; T parameter; Nu parameter; Ny parameter; Vdq output; Wyp parameter; Wup parameter; flux input; flux1 input; Vr input
function Vdq  = fcn(Wsl,Ir, Ir1,Iref,Ls, Lr, Rr, Lm, T, Nu, Ny, Wyp, Wup, flux,flux1,Vr)
assert (Ny <= 100);
assert (Nu <= 100);

%Variáveis auxiliares

Sigma = 1-Lm^2/(Ls*Lr);

%Entradas
eps = [Ir(1)-Ir1(1);Ir(2)-Ir1(2);Ir(1);Ir(2)];

dFlux=flux-flux1;
%Matrizes de estado discretizadas
A = [1-Rr*T/(Sigma*Lr),       Wsl*T;
          -Wsl*T,        1-Rr*T/(Sigma*Lr)];

B = [T/(Sigma*Lr),      0;
          0,        T/(Sigma*Lr)];
      
      
G = [          0,           Wsl*Lm*T/(Sigma*Ls*Lr);
      -Wsl*Lm*T/(Sigma*Ls*Lr),          0];
      
C = eye(2);


Aa=[A,zeros(2); C*A,eye(2)];

Ba = [B;C*B];

Ca = [zeros(2), eye(2)];

Ga = [G;C*G];
 
%Inicialização de matrizes
Ap = zeros(2*Ny,4);
Bp = zeros(2*Ny,2*Nu);

Refp = zeros(2*Ny,1);
Wdp = zeros(2*Ny,1);

Dp = zeros(2*Ny,2*Ny);


%Cálculo das matrizes
for i=1:Ny
    Ap((i-1)*2+1:i*2,1:4)= Ca*Aa^i;
    Refp((i-1)*2+1:i*2,1)=Iref;
    Wdp((i-1)*2+1:i*2,1)=[dFlux;0];
    for j=1:i
        if j<=Nu
            Bp((i-1)*2+1:i*2,(j-1)*2+1:j*2)=Ca*Aa^(i-j)*Ba;
        end
        Dp((i-1)*2+1:i*2,(j-1)*2+1:j*2)=Ca*Aa^(i-j)*Ga;
    end
end
%Minimização

dU = (Bp.'*Wyp*Bp+Wup)\(Bp.'*Wyp*(Refp-Ap*eps-Dp*Wdp));
% 164.3*Ird1 - 306.4*Ird + 142.1*Irefd - 0.0304*Irefq - 0.3686*Irq + 0.399*Irq1
%   36.95*Ird + 14.14*Ird1 - 51.09*Irefd + 93.76*Irefq - 229.9*Irq + 136.1*Irq1
Vdq = Vr + dU(1:2,1);

== matlab function dfig/MATLAB Function ==
  data: u input
function fcn(u)
%#codegen
coder.extrinsic('set_param')
coder.extrinsic('get_param')
if u>=0.2
    if strcmp(get_param('dfig/DFIG','Lm'),'Lm')
        while strcmp(get_param('dfig','SimulationStatus'),'running')
            set_param('dfig','SimulationCommand','pause'); % to pause simulation
        end
        disp(get_param('dfig','SimulationStatus'));
        if strcmp(get_param('dfig','SimulationStatus'),'paused')
            set_param('dfig/DFIG','Lm','Lm*(1+dLm/100)');
            set_param('dfig/DFIG','Rotor','[(Rr*(1+dRr/100)) (Lr-Lm)]');
            set_param('dfig','SimulationCommand','update');
            set_param('dfig','SimulationCommand','continue');
        end
    end
%    set_param('dfig','SimulationCommand','continue');
end
